simulink model "T6_bloques"  (R2025a)
settings: Solver=VariableStepAuto  StartTime=0.0  StopTime=0.002  RelTol=1e-3
InitFcn:
  | L = 2e-3;
  | R = 10;
  | C = 10e-6;
  | U = 32;
settings Model: Creator=carlo  LastModifiedBy=carlo

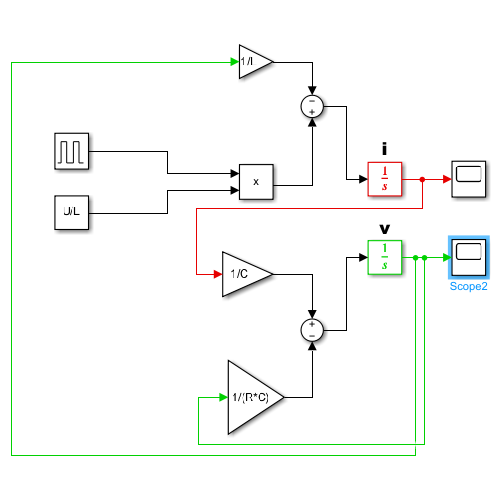
[thumbnail: Simulink's stored preview of the top-level diagram]
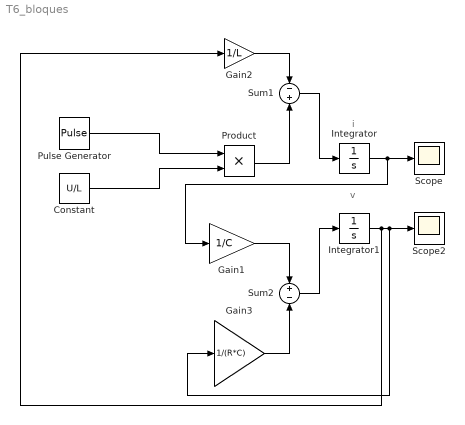
== system T6_bloques ==
  note: i
  note: v
  Constant : Constant  Value=U/L
  Gain1 : Gain  Gain=1/C
  Gain2 : Gain  Gain=1/L
  Gain3 : Gain  Gain=1/(R*C)
  Integrator : Integrator
  Integrator1 : Integrator
  Product : Product
  Pulse Generator : DiscretePulseGenerator  PulseType=Time based  Period=0.00001  PulseWidth=40
  Scope : Scope
      settings: ActiveDisplayYMinimum=1.3030509267266697  ActiveDisplayYMaximum=1.395731877493438  DataLoggingVariableName=ScopeData2
  Scope2 : Scope
      settings: ActiveDisplayYMinimum=-1.3028213286617349  ActiveDisplayYMaximum=14.593143629957261  DataLoggingVariableName=ScopeData3
  Sum1 : Sum  Inputs=-+
  Sum2 : Sum  Inputs=+-
  wires:
  Gain2/1 -> Sum1/1
  Sum1/1 -> Integrator/1
  Gain3/1 -> Sum2/2
  Sum2/1 -> Integrator1/1
  Integrator1/1 -> Gain2/1, Gain3/1, Scope2/1
  Integrator/1 -> Gain1/1, Scope/1
  Gain1/1 -> Sum2/1
  Product/1 -> Sum1/2
  Pulse Generator/1 -> Product/1
  Constant/1 -> Product/2
